simulink model "pentaNetMDL"  (R2014a)
settings: Solver=ode45  StartTime=0.0  StopTime=10.0  RelTol=1e-3
values from neighbouring files (symbols this model uses):
  A = -L    [pentaNet.m]
  C = eye(5)    [pentaNet.m]
  D = [-2 1 1 1 0 ... (first row only)    [pentaNet.m]
  f1Val = 10    [pentaNet.m]
  f2Val = 10    [pentaNet.m]
  f3Val = 10    [pentaNet.m]
  f4Val = 10    [pentaNet.m]
  f5Val = 10    [pentaNet.m]
  flt1 = 0    [pentaNet.m]
  flt2 = 1    [pentaNet.m]
  flt3 = 0    [pentaNet.m]
  flt4 = 1    [pentaNet.m]
  flt5 = 0    [pentaNet.m]
  L = Deg-Ag    [pentaNet.m]
  pCV = CV*inv(CV'*CV)*CV'    [pentaNet.m]
  tf1 = 12    [pentaNet.m]
  tf2 = 2    [pentaNet.m]
  tf3 = 1    [pentaNet.m]
  tf4 = 3    [pentaNet.m]
  tf5 = 4    [pentaNet.m]
  x0 = [0 1 1 0 0]    [pentaNet.m]
undefined symbols (not defined in the file or in its folder): magnitude
settings Model: Creator=sqn4594  LastModifiedBy=sqn4594

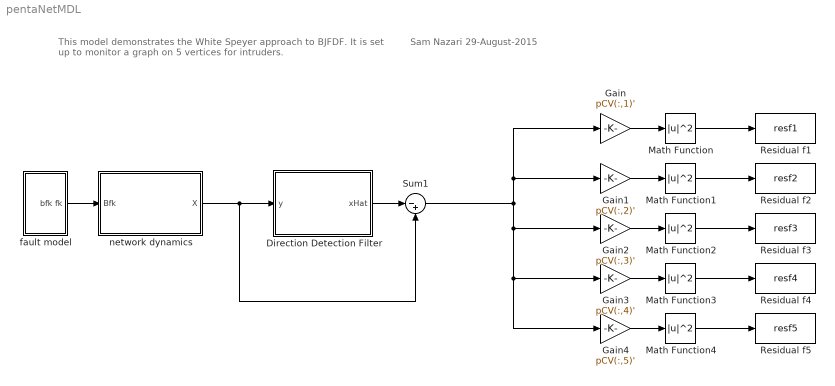
== system pentaNetMDL ==
  note: Sam Nazari
      | 29-August-2015
  note: This model demonstrates the White Speyer approach to BJFDF.
      | It is set up to monitor a graph on 5 vertices for intruders.
  Direction Detection Filter : Subsystem
  Gain : Gain  Gain=pCV(:,1)'
  Gain1 : Gain  Gain=pCV(:,2)'
  Gain2 : Gain  Gain=pCV(:,3)'
  Gain3 : Gain  Gain=pCV(:,4)'
  Gain4 : Gain  Gain=pCV(:,5)'
  Math Function{,1..4} (5 alike) : Math  Operator=magnitude^2  SaturateOnIntegerOverflow=on
  Residual f1 : ToWorkspace  VariableName=resf1  SampleTime=-1
  Residual f2 : ToWorkspace  VariableName=resf2  SampleTime=-1
  Residual f3 : ToWorkspace  VariableName=resf3  SampleTime=-1
  Residual f4 : ToWorkspace  VariableName=resf4  SampleTime=-1
  Residual f5 : ToWorkspace  VariableName=resf5  SampleTime=-1
  Sum1 : Sum  Inputs=|-+
  fault model : Subsystem
  network dynamics : Subsystem
  wires:
  fault model/1(bfk fk) -> network dynamics/1(Bfk)
  network dynamics/1(X) -> Sum1/2, Direction Detection Filter/1(y)
  Gain/1 -> Math Function/1
  Gain1/1 -> Math Function1/1
  Gain2/1 -> Math Function2/1
  Gain3/1 -> Math Function3/1
  Gain4/1 -> Math Function4/1
  Math Function/1 -> Residual f1/1
  Math Function1/1 -> Residual f2/1
  Math Function2/1 -> Residual f3/1
  Math Function3/1 -> Residual f4/1
  Math Function4/1 -> Residual f5/1
  Direction Detection Filter/1("xHat ") -> Sum1/1
  Sum1/1 -> Gain4/1, Gain3/1, Gain2/1, Gain/1, Gain1/1

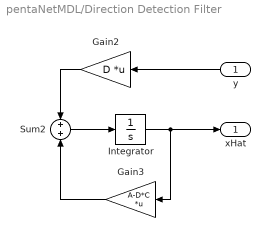
== system pentaNetMDL/Direction Detection Filter ==
  y : Inport
  Gain2 : Gain  Gain=D  Multiplication=Matrix(K*u)
  Gain3 : Gain  Gain=A-D*C  Multiplication=Matrix(K*u)
  Integrator : Integrator
  Sum2 : Sum
  "xHat " : Outport
  wires:
  y/1 -> Gain2/1
  Sum2/1 -> Integrator/1
  Integrator/1 -> "xHat "/1, Gain3/1
  Gain2/1 -> Sum2/1
  Gain3/1 -> Sum2/2

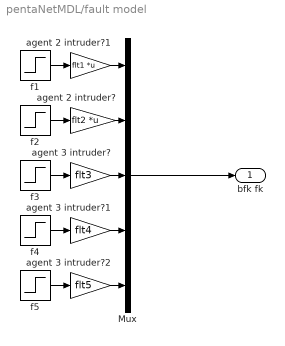
== system pentaNetMDL/fault model ==
  Mux : Mux  Inputs=5
  agent 2 intruder? : Gain  Gain=flt2  Multiplication=Matrix(K*u)
  agent 2 intruder?1 : Gain  Gain=flt1  Multiplication=Matrix(K*u)
  agent 3 intruder? : Gain  Gain=flt3
  agent 3 intruder?1 : Gain  Gain=flt4
  agent 3 intruder?2 : Gain  Gain=flt5
  f1 : Step  After=f1Val  SampleTime=tf1
  f2 : Step  After=f2Val  SampleTime=tf2
  f3 : Step  After=f3Val  SampleTime=tf3
  f4 : Step  After=f4Val  SampleTime=tf4
  f5 : Step  After=f5Val  SampleTime=tf5
  bfk fk : Outport
  wires:
  Mux/1 -> bfk fk/1
  f1/1 -> agent 2 intruder?1/1
  f2/1 -> agent 2 intruder?/1
  f3/1 -> agent 3 intruder?/1
  agent 2 intruder?/1 -> Mux/2
  agent 3 intruder?/1 -> Mux/3
  agent 2 intruder?1/1 -> Mux/1
  f4/1 -> agent 3 intruder?1/1
  agent 3 intruder?1/1 -> Mux/4
  agent 3 intruder?2/1 -> Mux/5
  f5/1 -> agent 3 intruder?2/1

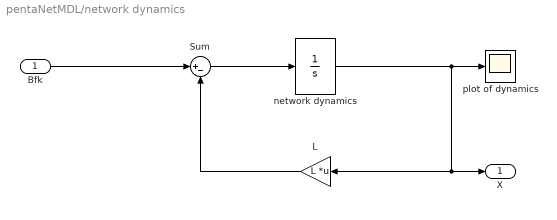
== system pentaNetMDL/network dynamics ==
  Bfk : Inport
  L : Gain  Gain=L  Multiplication=Matrix(K*u)
  Sum : Sum  Inputs=|+-
  network dynamics : Integrator  InitialCondition=x0
  plot of dynamics : Scope
  X : Outport
  wires:
  Bfk/1 -> Sum/1
  Sum/1 -> network dynamics/1
  network dynamics/1 -> plot of dynamics/1, X/1, L/1
  L/1 -> Sum/2
